simulink model "MPCSimulation"  (R2021b)
settings: Solver=VariableStepAuto  StartTime=0.0  StopTime=tsim  RelTol=1e-3  EnableMultiTasking=on
values from neighbouring files (symbols this model uses):
  C = [eye(4),zeros(4)]    [MPCController.m]    (also in setupsimulation.m)
  M = 3    [MPCController.m]    (also in setupsimulation.m; yalmip_mpc.m)
  Mu = params.l*params.Cfx*eye(nu)    [MPCController.m]    (also in setupsimulation.m)
  Muinv = Mu\eye(nu)    [MPCController.m]    (also in setupsimulation.m)
  Mxi = diag([sqrt(params.Cfx*params.l/params.m),                sqrt(params.Cfx*params.l/params.m),                1,                sqrt(params.Cfx/params.m/params.l)*ones(1,5)])    [MPCController.m]    (also in setupsimulation.m = diag([sqrt(params.Cfx*params.l/params.m),            sqrt(pa)
  Mxinv = Mxi\eye(nx)    [MPCController.m]    (also in setupsimulation.m)
  N = 10    [MPCController.m]    (also in setupsimulation.m; yalmip_mpc.m)
  nu = 4    [MPCController.m]    (also in setupsimulation.m; yalmip_mpc.m)
  nx = 8    [MPCController.m]    (also in setupsimulation.m; yalmip_mpc.m)
  ny = size(C,1)    [MPCController.m]    (also in setupsimulation.m)
  Ts = 0.05    [setupsimulation.m]    (also in yalmip_mpc.m)
  u0 = zeros(4,1)    [setupsimulation.m]
  xi0 = [0; vx0; 0; 0; 250/79*vx0*ones(4,1)]    [setupsimulation.m]
undefined symbols (not defined in the file or in its folder): odeSimulationModel, SimulationModel
settings Model: Creator=johanl  LastModifiedBy=PBM
settings SolverCC: AlgebraicLoopSolver=TrustRegion
settings DataIOCC: LimitDataPoints=on  SaveFormat=Array  SignalLoggingSaveFormat=ModelDataLogs  ReturnWorkspaceOutputs=off
settings OptimizationCC: ExpressionDepthLimit=2147483647  LifeSpan=inf
settings DebuggingCC: UnderspecifiedInitializationDetection=Classic  MergeDetectMultiDrivingBlocksExec=none  SolverPrmCheckMsg=warning  FcnCallInpInsideContextMsg=warning  StateNameClashWarn=warning  SFUnexpectedBacktrackingDiag=warning  SFNoUnconditionalDefaultTransitionDiag=warning  SFExecutionAtInitializationDiag=none  SFMachineParentedDataDiag=warning  ArithmeticOperatorsInVariantConditions=warning
settings HardwareCC: ProdBitPerPointer=32  ProdBitPerSizeT=32  ProdBitPerPtrDiffT=32  ProdLargestAtomicFloat=None  ProdIntDivRoundTo=Undefined  ProdEndianess=Unspecified  ProdWordSize=32  ProdHWDeviceType=32-bit Generic
settings ModelReferenceCC: PropagateSignalLabelsOutOfModel=off
settings SFSimCC: SimUseLocalCustomCode=off  CustomCodeUndefinedFunction=UseInterfaceOnly
settings RTWCC: RTWUseLocalCustomCode=off
settings CodeAppCC: StateflowObjectComments=on
settings GRTTargetCC: TargetLangStandard=C89/C90 (ANSI)
settings ConfigComp: CovMetricSettings=dw  CovSaveCumulativeToWorkspaceVar=on  CovSaveSingleToWorkspaceVar=on  CovExternalEMLEnable=off

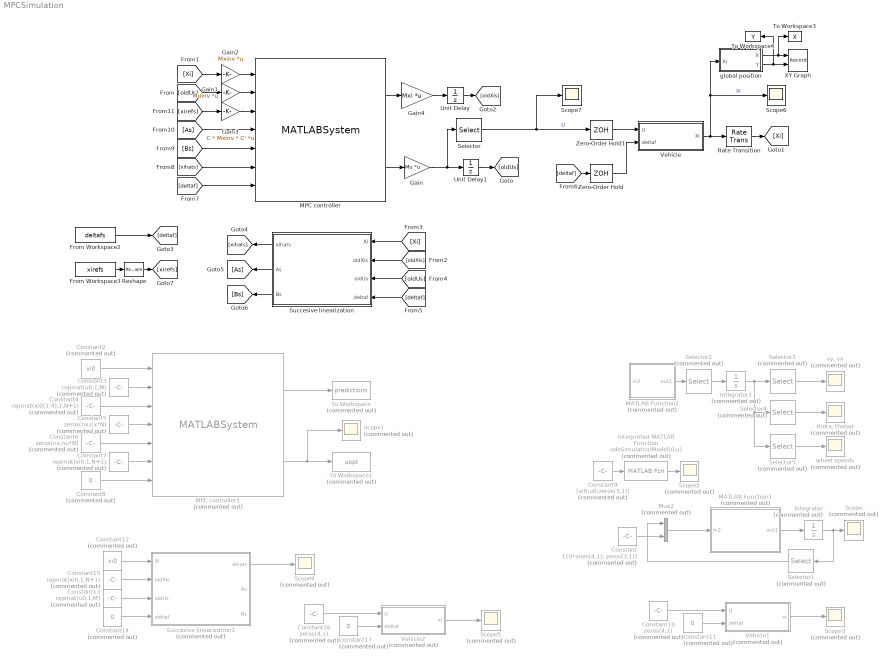
== system MPCSimulation ==
  Constant : Constant  Commented=on  Value=[10*ones(4,1); zeros(3,1)]
  Constant10 : Constant  Commented=on  Value=zeros(4,1)  SampleTime=Ts
  Constant{8,11,14,17} (4 alike) : Constant  Commented=on  Value=0
  Constant12 : Constant  Commented=on  Value=xi0  SampleTime=Ts
  Constant13 : Constant  Commented=on  Value=repmat(u0,1,M)
  Constant15 : Constant  Commented=on  Value=repmat(xi0,1,N+1)
  Constant16 : Constant  Commented=on  Value=zeros(4,1)  SampleTime=Ts
  Constant2 : Constant  Commented=on  Value=xi0  SampleTime=Ts
  Constant3 : Constant  Commented=on  Value=repmat(u0,1,M)
  Constant4 : Constant  Commented=on  Value=repmat(xi0(1:4),1,N+1)
  Constant5 : Constant  Commented=on  Value=zeros(nx,nx*N)
  Constant6 : Constant  Commented=on  Value=zeros(nx,nu*N)
  Constant7 : Constant  Commented=on  Value=repmat(xi0,1,N+1)
  Constant9 : Constant  Commented=on  Value=[xi0;u0;zeros(3,1)]
  From Workspace2 : FromWorkspace  VariableName=deltafs  SampleTime=Ts  OutputAfterFinalValue=Holding final value
  From Workspace3 : FromWorkspace  VariableName=xirefs  SampleTime=Ts  OutputAfterFinalValue=Holding final value
  Gain : Gain  Gain=Mu  Multiplication=Matrix(K*u)
  Gain1 : Gain  Gain=Muinv  Multiplication=Matrix(K*u)
  Gain2 : Gain  Gain=Mxinv  Multiplication=Matrix(K*u)
  Gain3 : Gain  Gain=C * Mxinv * C'  Multiplication=Matrix(K*u)
  Gain4 : Gain  Gain=Mxi  Multiplication=Matrix(K*u)
  Integrator : Integrator  Commented=on  InitialCondition=[0; 10; 0; 0; 250/79*10*ones(4,1);zeros(7,1)];
  Integrator1 : Integrator  Commented=on  InitialCondition=[0; 10; 0; 0; 250/79*10*ones(4,1);zeros(7,1)];
  Interpreted MATLAB Function : MATLABFcn  Commented=on  MATLABFcn=odeSimulationModel(0,u)
  MATLAB Function1 : MATLAB Function  Commented=on  TreatAsAtomicUnit=on
  MATLAB Function2 : MATLAB Function  Commented=on  TreatAsAtomicUnit=on
  MPC controller : MATLABSystem  System=yalmip_mpc  nx=nx  nu=nu  N=N  M=M  Ts=Ts  SimulateUsing=Interpreted execution
      mask Type: yalmip_mpc
      mask Display:
      | disp('yalmip_mpc');
      | port_label('input',1,'Xi');
      | port_label('input',2,'oldUs');
      | port_label('input',3,'xirefs');
      | port_label('input',4,'As');
      | port_label('input',5,'Bs');
      | port_label('input',6,'xihats');
      | port_label('input',7,'deltaf');
      | port_label('output',1,'predictions');
      | port_label('output',2,'uopt');
  MPC controller1 : MATLABSystem  Commented=on  System=yalmip_mpc  nx=nx  nu=nu  N=N  M=M  Ts=Ts  SimulateUsing=Interpreted execution
      mask Type: yalmip_mpc
      mask Display:
      | disp('yalmip_mpc');
      | port_label('input',1,'Xi');
      | port_label('input',2,'oldUs');
      | port_label('input',3,'xirefs');
      | port_label('input',4,'As');
      | port_label('input',5,'Bs');
      | port_label('input',6,'xihats');
      | port_label('input',7,'deltaf');
      | port_label('output',1,'predictions');
      | port_label('output',2,'uopt');
  Mux2 : Mux  Commented=on  Inputs=2
  Rate Transition : RateTransition  InitialCondition=xi0  OutPortSampleTime=Ts
  Reshape : Reshape  OutputDimensionality=Customize  OutputDimensions=[ny,N+1]
  Scope{,1..5} (6 alike) : Scope  Commented=on
  Scope6 : Scope
  Scope7 : Scope
  Selector : Selector  NumberOfDimensions=2  InputPortWidth=3  IndexOptions=Index vector (dialog),Index vector (dialog)  Indices=1:nu,1  OutputSizes=1,1
  Selector1 : Selector  Commented=on  InputPortWidth=15  IndexOptions=Index vector (dialog)  Indices=[1:8]  OutputSizes=1
  Selector2 : Selector  Commented=on  InputPortWidth=15  IndexOptions=Index vector (dialog)  Indices=[1:8]  OutputSizes=1
  Selector3 : Selector  Commented=on  InputPortWidth=8  IndexOptions=Index vector (dialog)  Indices=[1:2]  OutputSizes=1
  Selector4 : Selector  Commented=on  InputPortWidth=8  IndexOptions=Index vector (dialog)  Indices=[3:4]  OutputSizes=1
  Selector5 : Selector  Commented=on  InputPortWidth=8  IndexOptions=Index vector (dialog)  Indices=[5:8]  OutputSizes=1
  Succesive linearization : MATLAB Function  TreatAsAtomicUnit=on
  Succesive linearization1 : MATLAB Function  Commented=on  TreatAsAtomicUnit=on
  To Workspace : ToWorkspace  Commented=on  VariableName=predictions  SaveFormat=Timeseries  SampleTime=-1
  To Workspace1 : ToWorkspace  Commented=on  VariableName=uopt  SaveFormat=Timeseries  SampleTime=-1
  To Workspace3 : ToWorkspace  VariableName=X  SampleTime=-1
  To Workspace4 : ToWorkspace  VariableName=Y  SampleTime=-1
  Unit Delay : UnitDelay  InitialCondition=repmat(xi0,1,N+1)  SampleTime=-1  HasFrameUpgradeWarning=on
  Unit Delay1 : UnitDelay  InitialCondition=repmat(u0,1,M)  SampleTime=-1  HasFrameUpgradeWarning=on
  Vehicle : Subsystem
  Vehicle1 : Subsystem  Commented=on
  Vehicle2 : Subsystem  Commented=on
  XY Graph : Record  FileSettingsInternal="{\"entries\":[{\"content\":{\"excelSettings\":{\"content\":{},\"type\":\"Streamout.ExcelSettings\"}},\"type\":\"Streamout.FileSettingStorage\",\"uuid\":\"9bd8e3e6-cf03-4281-bd11-05e1fe8b1948\"}],\"packageUris\":[\"http://schema.mathworks.com/mf0/streamout_blocks/R2020a\"],\"version\":\"1.0\"}"  Layout=[1 1]  SignalsInternal="{\"entries\":[{\"content\":{\"signals\":[{\"content\":{\"blockPath\":[\"MPCSimulation/XY Graph\"],\"channel\":[],\"dimensions\":[1],\"domain\":\"MPCSimulation/XY Graph\",\"lineColor\":\"#a2142f\",\"plots\":[1],\"port\":1,\"sid\":[],\"signalID\":53,\"signalName\":\"XY Graph:1\"},\"type\":\"RecordBlkView.Signal\",\"uuid\":\"acc0aba6-a077-4c69-b4eb-e56c431fcc30\"},{\"content\":{\"blockPath\":[\"MPCSimulation/XY Graph\"],\"channel\":[],\"dimensions\":[1],\"domain\":\"MPCSimulation/XY Graph\",\"lineColor\":\"#139fff\",\"plots\":[1],\"port\":2,\"sid\":[],\"signalID\":56,\"signalName\":\"XY Graph:2\"},\"type\":\"RecordBlkView.Signal\",\"uuid\":\"2464f634-715d-4349-a932-ac5f9f95b442\"}]},\"type\":\"RecordBlkView.InputSignals\",\"uuid\":\"c07f4d52-6f61-44b7-b332-b508ada1f36c\"}],\"packageUris\":[\"http://schema.mathworks.com/mf0/streamout_blocks/R2020a\"],\"version\":\"1.0\"}"  VisualizationBindings="{\"xyplotplugin\":{\"info\":[{\"series\":[{\"bindingParametersList\":[{\"parameter\":\"X-Axis\",\"signalID\":53,\"signalName\":\"XY Graph:1\"},{\"parameter\":\"Y-Axis\",\"signalID\":56,\"signalName\":\"XY Graph:2\"}],\"seriesID\":48449}],\"subplotID\":1}]}}"  CompatibilityTag=XY  st=-1
  Zero-Order Hold : ZeroOrderHold  SampleTime=Ts
  Zero-Order Hold1 : ZeroOrderHold  SampleTime=Ts
  global position : Subsystem
  "theta, thetad" : Scope  Commented=on
  "vy, vx" : Scope  Commented=on
  wheel speeds : Scope  Commented=on
  wires:
  Integrator1/1 -> Selector5/1, Selector4/1, Selector3/1
  Mux2/1 -> MATLAB Function1/1(in2)
  MATLAB Function1/1(out1) -> Integrator/1
  Integrator/1 -> Selector1/1, Scope/1
  Constant/1 -> Mux2/2
  Selector1/1 -> Mux2/1
  MATLAB Function2/1(out1) -> Selector2/1
  Selector2/1 -> Integrator1/1
  Selector3/1 -> "vy, vx"/1
  Selector4/1 -> "theta, thetad"/1
  Selector5/1 -> wheel speeds/1
  Constant2/1 -> MPC controller1/1
  Constant3/1 -> MPC controller1/2
  Constant4/1 -> MPC controller1/3
  Constant5/1 -> MPC controller1/4
  Constant6/1 -> MPC controller1/5
  Constant7/1 -> MPC controller1/6
  Constant8/1 -> MPC controller1/7
  MPC controller1/1 -> To Workspace/1
  MPC controller1/2 -> Scope1/1, To Workspace1/1
  Constant9/1 -> Interpreted MATLAB Function/1
  Interpreted MATLAB Function/1 -> Scope2/1
  Selector/1 -> Scope7/1, Zero-Order Hold1/1  "U"
  [Xi] -> Gain2/1
  [deltaf] -> Succesive linearization/4(deltaf)
  [deltaf] -> Zero-Order Hold/1
  [deltaf] -> MPC controller/7
  Succesive linearization/1(xihats) -> [xihats]
  Succesive linearization/2(As) -> [As]
  [Bs] -> MPC controller/5
  Succesive linearization/3(Bs) -> [Bs]
  [xihats] -> MPC controller/6
  [As] -> MPC controller/4
  From Workspace2/1 -> [deltaf]
  [xirefs] -> Gain3/1
  Gain/1 -> Unit Delay1/1, Selector/1
  Gain1/1 -> MPC controller/2
  Gain2/1 -> MPC controller/1
  Gain3/1 -> MPC controller/3
  MPC controller/1 -> Gain4/1
  Gain4/1 -> Unit Delay/1
  [oldUs] -> Gain1/1
  MPC controller/2 -> Gain/1
  From Workspace3/1 -> Reshape/1
  Reshape/1 -> [xirefs]
  Constant10/1 -> Vehicle1/1(U)
  Constant11/1 -> Vehicle1/2(deltaf)
  Vehicle1/1(xi) -> Scope3/1
  Constant12/1 -> Succesive linearization1/1(Xi)
  Constant13/1 -> Succesive linearization1/3(oldUs)
  Constant14/1 -> Succesive linearization1/4(deltaf)
  Constant15/1 -> Succesive linearization1/2(oldXis)
  Succesive linearization1/1(xihats) -> Scope4/1
  Vehicle2/1(xi) -> Scope5/1
  Constant17/1 -> Vehicle2/2(deltaf)
  Constant16/1 -> Vehicle2/1(U)
  Vehicle/1(Xi) -> global position/1(Xi), Scope6/1, Rate Transition/1  "Xi"
  Zero-Order Hold/1 -> Vehicle/2(deltaf)
  Zero-Order Hold1/1 -> Vehicle/1(U)
  [Xi] -> Succesive linearization/1(Xi)
  Rate Transition/1 -> [Xi]
  [oldXis] -> Succesive linearization/2(oldXis)
  [oldUs] -> Succesive linearization/3(oldUs)
  Unit Delay1/1 -> [oldUs]
  Unit Delay/1 -> [oldXis]
  global position/1(X) -> To Workspace3/1, XY Graph/1
  global position/2(Y) -> To Workspace4/1, XY Graph/2

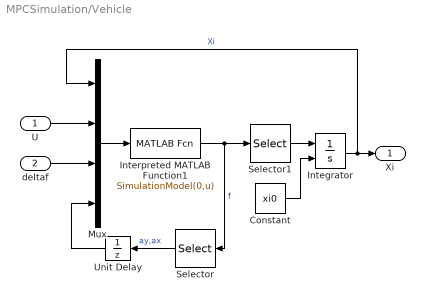
== system MPCSimulation/Vehicle ==
  U : Inport
  deltaf : Inport  Port=2
  Constant : Constant  Value=xi0
  Integrator : Integrator  InitialConditionSource=external  InitialCondition=xi0
  Interpreted MATLAB Function1 : MATLABFcn  MATLABFcn=SimulationModel(0,u)
  Mux : Mux
  Selector : Selector  IndexOptions=Index vector (dialog)  Indices=[1 2]  OutputSizes=1
  Selector1 : Selector  InputPortWidth=15  IndexOptions=Index vector (dialog)  Indices=[1:8]  OutputSizes=1
  Unit Delay : UnitDelay  InitialCondition=[0;0]  SampleTime=-1  HasFrameUpgradeWarning=on
  Xi : Outport  VectorParamsAs1DForOutWhenUnconnected=off
  wires:
  Interpreted MATLAB Function1/1 -> Selector/1, Selector1/1  "f"
  Constant/1 -> Integrator/2
  Integrator/1 -> Mux/1, Xi/1  "Xi"
  Mux/1 -> Interpreted MATLAB Function1/1
  U/1 -> Mux/2
  deltaf/1 -> Mux/3
  Selector1/1 -> Integrator/1
  Selector/1 -> Unit Delay/1  "ay,ax"
  Unit Delay/1 -> Mux/4

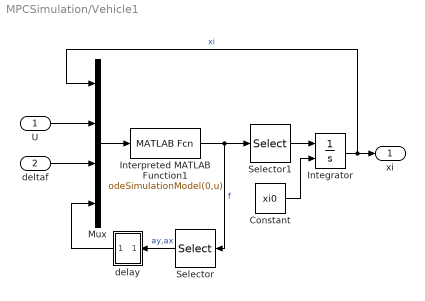
== system MPCSimulation/Vehicle1 ==
  U : Inport
  deltaf : Inport  Port=2
  Constant : Constant  Value=xi0
  Integrator : Integrator  InitialConditionSource=external  InitialCondition=xi0
  Interpreted MATLAB Function1 : MATLABFcn  MATLABFcn=odeSimulationModel(0,u)
  Mux : Mux
  Selector : Selector  IndexOptions=Index vector (dialog)  Indices=[1 2]  OutputSizes=1
  Selector1 : Selector  InputPortWidth=15  IndexOptions=Index vector (dialog)  Indices=[1:8]  OutputSizes=1
  delay : Subsystem
  xi : Outport  VectorParamsAs1DForOutWhenUnconnected=off
  wires:
  Interpreted MATLAB Function1/1 -> Selector/1, Selector1/1  "f"
  Constant/1 -> Integrator/2
  Integrator/1 -> Mux/1, xi/1  "xi"
  Mux/1 -> Interpreted MATLAB Function1/1
  U/1 -> Mux/2
  deltaf/1 -> Mux/3
  Selector1/1 -> Integrator/1
  Selector/1 -> delay/1(" ")  "ay,ax"
  delay/1(Out1) -> Mux/4

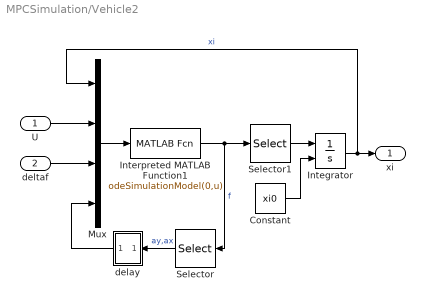
== system MPCSimulation/Vehicle2 ==
  U : Inport
  deltaf : Inport  Port=2
  Constant : Constant  Value=xi0
  Integrator : Integrator  InitialConditionSource=external  InitialCondition=xi0
  Interpreted MATLAB Function1 : MATLABFcn  MATLABFcn=odeSimulationModel(0,u)
  Mux : Mux
  Selector : Selector  IndexOptions=Index vector (dialog)  Indices=[1 2]  OutputSizes=1
  Selector1 : Selector  InputPortWidth=15  IndexOptions=Index vector (dialog)  Indices=[1:8]  OutputSizes=1
  delay : Subsystem
  xi : Outport  VectorParamsAs1DForOutWhenUnconnected=off
  wires:
  Interpreted MATLAB Function1/1 -> Selector/1, Selector1/1  "f"
  Constant/1 -> Integrator/2
  Integrator/1 -> Mux/1, xi/1  "xi"
  Mux/1 -> Interpreted MATLAB Function1/1
  U/1 -> Mux/2
  deltaf/1 -> Mux/3
  Selector1/1 -> Integrator/1
  Selector/1 -> delay/1(" ")  "ay,ax"
  delay/1(Out1) -> Mux/4

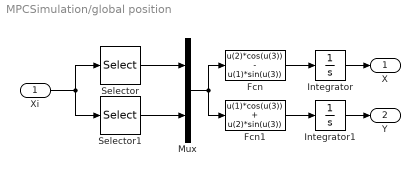
== system MPCSimulation/global position ==
  Xi : Inport
  Fcn : Fcn  Expr=u(2)*cos(u(3)) - u(1)*sin(u(3))
  Fcn1 : Fcn  Expr=u(1)*cos(u(3)) + u(2)*sin(u(3))
  Integrator : Integrator
  Integrator1 : Integrator
  Mux : Mux  Inputs=2
  Selector : Selector  InputPortWidth=8  IndexOptions=Index vector (dialog)  Indices=[1 2]  OutputSizes=1
  Selector1 : Selector  InputPortWidth=8  IndexOptions=Index vector (dialog)  Indices=3  OutputSizes=1
  X : Outport  VectorParamsAs1DForOutWhenUnconnected=off
  Y : Outport  Port=2  VectorParamsAs1DForOutWhenUnconnected=off
  wires:
  Xi/1 -> Selector1/1, Selector/1
  Selector/1 -> Mux/1
  Selector1/1 -> Mux/2
  Fcn/1 -> Integrator/1
  Mux/1 -> Fcn1/1, Fcn/1
  Fcn1/1 -> Integrator1/1
  Integrator/1 -> X/1
  Integrator1/1 -> Y/1

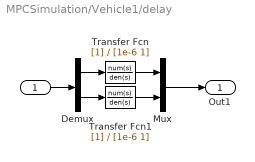
== system MPCSimulation/Vehicle1/delay ==
  " " : Inport
  Demux : Demux  Outputs=2
  Mux : Mux  Inputs=2
  Transfer Fcn : TransferFcn  Denominator=[1e-6 1]
  Transfer Fcn1 : TransferFcn  Denominator=[1e-6 1]
  Out1 : Outport  VectorParamsAs1DForOutWhenUnconnected=off
  wires:
  " "/1 -> Demux/1
  Demux/1 -> Transfer Fcn/1
  Demux/2 -> Transfer Fcn1/1
  Transfer Fcn1/1 -> Mux/2
  Transfer Fcn/1 -> Mux/1
  Mux/1 -> Out1/1

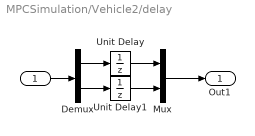
== system MPCSimulation/Vehicle2/delay ==
  " " : Inport
  Demux : Demux  Outputs=2
  Mux : Mux  Inputs=2
  Unit Delay : UnitDelay  SampleTime=-1  HasFrameUpgradeWarning=on
  Unit Delay1 : UnitDelay  SampleTime=-1  HasFrameUpgradeWarning=on
  Out1 : Outport  VectorParamsAs1DForOutWhenUnconnected=off
  wires:
  " "/1 -> Demux/1
  Demux/1 -> Unit Delay/1
  Unit Delay1/1 -> Mux/2
  Unit Delay/1 -> Mux/1
  Mux/1 -> Out1/1
  Demux/2 -> Unit Delay1/1

== matlab function MPCSimulation/MATLAB Function1 ==
  data: in2 input; out1 output
function out1 = odeSimulationModel(in2)
%ODESIMULATIONMODEL
%    OUT1 = ODESIMULATIONMODEL(TS,IN2)

%    This function was generated by the Symbolic Math Toolbox version 8.2.
%    15-Jan-2021 11:04:04

Mp_FL = in2(9,:);
Mp_FR = in2(10,:);
Mp_RL = in2(11,:);
Mp_RR = in2(12,:);
acc_lat_ms2 = in2(14,:);
acc_long_ms2 = in2(15,:);
steer_angle_FL = in2(13,:);
vx = in2(2,:);
vy = in2(1,:);
w_FL = in2(5,:);
w_FR = in2(6,:);
w_RL = in2(7,:);
w_RR = in2(8,:);
yaw_rate = in2(4,:);
t3 = vx.^2;
t6 = acc_lat_ms2.*2.41734219269103e2;
t7 = acc_long_ms2.*1.700046728971963e2;
t8 = t3.*4.29477476635514e-2;
t2 = -t6+t7+t8+3.28635e3;
t77 = yaw_rate.*(3.21e2./2.0e2);
t4 = -t77+vy;
t5 = acc_long_ms2.*5.219143457943925e3;
t9 = t6+t7+t8+3.28635e3;
t10 = t3.*1.318495853271028;
t11 = cos(steer_angle_FL);
t18 = yaw_rate.*7.585e-1;
t12 = -t18+vx;
t13 = t11.*t12;
t14 = sin(steer_angle_FL);
t15 = yaw_rate.*(1.07e2./1.0e2);
t16 = t15+vy;
t17 = t14.*t16;
t19 = t13+t17;
t20 = 1.0./t19;
t39 = w_FL.*(7.9e1./2.5e2);
t21 = t13+t17-t39;
t22 = t18+vx;
t23 = t11.*t22;
t24 = t17+t23;
t25 = 1.0./t24;
t47 = w_FR.*(7.9e1./2.5e2);
t26 = t17+t23-t47;
t27 = acc_lat_ms2.*3.597330257086355e2;
t28 = t7+t8+t27-4.929524999999999e3;
t29 = acc_lat_ms2.*1.104380388925511e4;
t30 = t7+t8-t27-4.929524999999999e3;
t31 = yaw_rate.*(3.01e2./4.0e2);
t32 = t31+vx;
t33 = 1.0./t32;
t62 = w_RR.*(7.9e1./2.5e2);
t34 = t31-t62+vx;
t35 = t31-vx;
t36 = 1.0./t35;
t37 = w_RL.*(7.9e1./2.5e2);
t38 = t31+t37-vx;
t40 = t20.*t21.*3.607731511888605;
t41 = atan(t40);
t42 = t41.*4.0;
t82 = t20.*t21.*1.803865755944303e1;
t43 = t42-t82;
t44 = atan(t43);
t45 = t44.*(2.9e1./2.0e1);
t46 = sin(t45);
t48 = t25.*t26.*3.607731511888605;
t49 = atan(t48);
t50 = t49.*4.0;
t83 = t25.*t26.*1.803865755944303e1;
t51 = t50-t83;
t52 = atan(t51);
t53 = t52.*(2.9e1./2.0e1);
t54 = sin(t53);
t55 = t11.*t16;
t56 = t12.*t14;
t57 = t28.^2;
t58 = t57.*2.35e-3;
t59 = t5+t10+t29+t58-1.513364175e5;
t85 = t14.*t22;
t60 = t55-t85;
t61 = t7+t8-t27-4.929524999999999e3;
t63 = t33.*t34.*3.607731511888605;
t64 = atan(t63);
t65 = t64.*4.0;
t66 = t65-t33.*t34.*1.803865755944303e1;
t67 = atan(t66);
t68 = t67.*(2.9e1./2.0e1);
t69 = sin(t68);
t88 = t36.*t38.*3.607731511888605;
t70 = atan(-t88);
t71 = t70.*4.0;
t72 = t36.*t38.*1.803865755944303e1;
t73 = t71+t72;
t74 = atan(t73);
t75 = t74.*(2.9e1./2.0e1);
t76 = sin(t75);
t78 = acc_lat_ms2.*7.421240531561462e3;
t79 = t2.^2;
t80 = t9.^2;
t81 = t5+t10+t78-t80.*2.35e-3+1.00890945e5;
t84 = t55-t56;
t86 = t7+t8-t27-4.929524999999999e3;
t87 = t7+t8-t27-4.929524999999999e3;
t89 = t2.*t76.*(7.9e1./2.5e2);
t90 = Mp_RL+t89;
out1 = [-vx.*yaw_rate-(t14.*t54.*(t7+t8-t27-4.929524999999999e3))./1.675e3-(t4.*(acc_lat_ms2.*(-7.421240531561462e3)+t5+t10-t79.*2.35e-3+1.00890945e5))./(vx.*1.675e3-yaw_rate.*1.2604375e3)-(t14.*t28.*t46)./1.675e3-(t4.*t33.*t81)./1.675e3+(t11.*t25.*t60.*(t5+t10-t29+t30.^2.*2.35e-3-1.513364175e5))./1.675e3-(t11.*t20.*t59.*(t56-t11.*t16))./1.675e3;t3.*(-2.526268656716418e-4)-(t2.*t76)./1.675e3+(t9.*t69)./1.675e3+vy.*yaw_rate-(t11.*t28.*t46)./1.675e3-(t11.*t30.*t54)./1.675e3-(t14.*t20.*t59.*t84)./1.675e3-(t14.*t25.*t60.*(t5+t10-t29+t61.^2.*2.35e-3-1.513364175e5))./1.675e3;yaw_rate;t2.*t76.*2.875429881543752e-4+t9.*t69.*2.875429881543752e-4+t11.*t28.*t46.*2.898356897210546e-4-t14.*t28.*t46.*4.088651127244937e-4-t11.*t30.*t54.*2.898356897210546e-4-t14.*t30.*t54.*4.088651127244937e-4+t4.*t33.*t81.*6.132976690867405e-4-t4.*t36.*(t5+t10-t78-t79.*2.35e-3+1.00890945e5).*6.132976690867405e-4+t11.*t20.*t59.*t84.*4.088651127244937e-4+t14.*t20.*t59.*t84.*2.898356897210546e-4+t11.*t25.*t60.*(t5+t10-t29+t86.^2.*2.35e-3-1.513364175e5).*4.088651127244937e-4-t14.*t25.*t60.*(t5+t10-t29+t87.^2.*2.35e-3-1.513364175e5).*2.898356897210546e-4;Mp_FL+t28.*t46.*(7.9e1./2.5e2);Mp_FR+t54.*(t7+t8-t27-4.929524999999999e3).*(7.9e1./2.5e2);t90;t90;Mp_FL;Mp_FR;Mp_RL;Mp_RR;steer_angle_FL;acc_lat_ms2;acc_long_ms2];
end

== matlab function MPCSimulation/MATLAB Function2 ==
  data: in2 input; out1 output
function out1 = odeSimulationModel(in2)
%ODESIMULATIONMODEL
%    OUT1 = ODESIMULATIONMODEL(TS,IN2)

%    This function was generated by the Symbolic Math Toolbox version 8.2.
%    15-Jan-2021 11:04:04

Mp_FL = in2(9,:);
Mp_FR = in2(10,:);
Mp_RL = in2(11,:);
Mp_RR = in2(12,:);
acc_lat_ms2 = in2(14,:);
acc_long_ms2 = in2(15,:);
steer_angle_FL = in2(13,:);
vx = in2(2,:);
vy = in2(1,:);
w_FL = in2(5,:);
w_FR = in2(6,:);
w_RL = in2(7,:);
w_RR = in2(8,:);
yaw_rate = in2(4,:);
t3 = vx.^2;
t6 = acc_lat_ms2.*2.41734219269103e2;
t7 = acc_long_ms2.*1.700046728971963e2;
t8 = t3.*4.29477476635514e-2;
t2 = -t6+t7+t8+3.28635e3;
t77 = yaw_rate.*(3.21e2./2.0e2);
t4 = -t77+vy;
t5 = acc_long_ms2.*5.219143457943925e3;
t9 = t6+t7+t8+3.28635e3;
t10 = t3.*1.318495853271028;
t11 = cos(steer_angle_FL);
t18 = yaw_rate.*7.585e-1;
t12 = -t18+vx;
t13 = t11.*t12;
t14 = sin(steer_angle_FL);
t15 = yaw_rate.*(1.07e2./1.0e2);
t16 = t15+vy;
t17 = t14.*t16;
t19 = t13+t17;
t20 = 1.0./t19;
t39 = w_FL.*(7.9e1./2.5e2);
t21 = t13+t17-t39;
t22 = t18+vx;
t23 = t11.*t22;
t24 = t17+t23;
t25 = 1.0./t24;
t47 = w_FR.*(7.9e1./2.5e2);
t26 = t17+t23-t47;
t27 = acc_lat_ms2.*3.597330257086355e2;
t28 = t7+t8+t27-4.929524999999999e3;
t29 = acc_lat_ms2.*1.104380388925511e4;
t30 = t7+t8-t27-4.929524999999999e3;
t31 = yaw_rate.*(3.01e2./4.0e2);
t32 = t31+vx;
t33 = 1.0./t32;
t62 = w_RR.*(7.9e1./2.5e2);
t34 = t31-t62+vx;
t35 = t31-vx;
t36 = 1.0./t35;
t37 = w_RL.*(7.9e1./2.5e2);
t38 = t31+t37-vx;
t40 = t20.*t21.*3.607731511888605;
t41 = atan(t40);
t42 = t41.*4.0;
t82 = t20.*t21.*1.803865755944303e1;
t43 = t42-t82;
t44 = atan(t43);
t45 = t44.*(2.9e1./2.0e1);
t46 = sin(t45);
t48 = t25.*t26.*3.607731511888605;
t49 = atan(t48);
t50 = t49.*4.0;
t83 = t25.*t26.*1.803865755944303e1;
t51 = t50-t83;
t52 = atan(t51);
t53 = t52.*(2.9e1./2.0e1);
t54 = sin(t53);
t55 = t11.*t16;
t56 = t12.*t14;
t57 = t28.^2;
t58 = t57.*2.35e-3;
t59 = t5+t10+t29+t58-1.513364175e5;
t85 = t14.*t22;
t60 = t55-t85;
t61 = t7+t8-t27-4.929524999999999e3;
t63 = t33.*t34.*3.607731511888605;
t64 = atan(t63);
t65 = t64.*4.0;
t66 = t65-t33.*t34.*1.803865755944303e1;
t67 = atan(t66);
t68 = t67.*(2.9e1./2.0e1);
t69 = sin(t68);
t88 = t36.*t38.*3.607731511888605;
t70 = atan(-t88);
t71 = t70.*4.0;
t72 = t36.*t38.*1.803865755944303e1;
t73 = t71+t72;
t74 = atan(t73);
t75 = t74.*(2.9e1./2.0e1);
t76 = sin(t75);
t78 = acc_lat_ms2.*7.421240531561462e3;
t79 = t2.^2;
t80 = t9.^2;
t81 = t5+t10+t78-t80.*2.35e-3+1.00890945e5;
t84 = t55-t56;
t86 = t7+t8-t27-4.929524999999999e3;
t87 = t7+t8-t27-4.929524999999999e3;
t89 = t2.*t76.*(7.9e1./2.5e2);
t90 = Mp_RL+t89;
out1 = [-vx.*yaw_rate-(t14.*t54.*(t7+t8-t27-4.929524999999999e3))./1.675e3-(t4.*(acc_lat_ms2.*(-7.421240531561462e3)+t5+t10-t79.*2.35e-3+1.00890945e5))./(vx.*1.675e3-yaw_rate.*1.2604375e3)-(t14.*t28.*t46)./1.675e3-(t4.*t33.*t81)./1.675e3+(t11.*t25.*t60.*(t5+t10-t29+t30.^2.*2.35e-3-1.513364175e5))./1.675e3-(t11.*t20.*t59.*(t56-t11.*t16))./1.675e3;t3.*(-2.526268656716418e-4)-(t2.*t76)./1.675e3+(t9.*t69)./1.675e3+vy.*yaw_rate-(t11.*t28.*t46)./1.675e3-(t11.*t30.*t54)./1.675e3-(t14.*t20.*t59.*t84)./1.675e3-(t14.*t25.*t60.*(t5+t10-t29+t61.^2.*2.35e-3-1.513364175e5))./1.675e3;yaw_rate;t2.*t76.*2.875429881543752e-4+t9.*t69.*2.875429881543752e-4+t11.*t28.*t46.*2.898356897210546e-4-t14.*t28.*t46.*4.088651127244937e-4-t11.*t30.*t54.*2.898356897210546e-4-t14.*t30.*t54.*4.088651127244937e-4+t4.*t33.*t81.*6.132976690867405e-4-t4.*t36.*(t5+t10-t78-t79.*2.35e-3+1.00890945e5).*6.132976690867405e-4+t11.*t20.*t59.*t84.*4.088651127244937e-4+t14.*t20.*t59.*t84.*2.898356897210546e-4+t11.*t25.*t60.*(t5+t10-t29+t86.^2.*2.35e-3-1.513364175e5).*4.088651127244937e-4-t14.*t25.*t60.*(t5+t10-t29+t87.^2.*2.35e-3-1.513364175e5).*2.898356897210546e-4;Mp_FL+t28.*t46.*(7.9e1./2.5e2);Mp_FR+t54.*(t7+t8-t27-4.929524999999999e3).*(7.9e1./2.5e2);t90;t90;Mp_FL;Mp_FR;Mp_RL;Mp_RR;steer_angle_FL;acc_lat_ms2;acc_long_ms2];
end

== matlab function MPCSimulation/Succesive linearization ==
  settings: updateMethod=DISCRETE  sampleTime=Ts
  data: Xi input; xihats output; oldXis input; oldUs input; deltaf input; As output; Bs output; MPCData parameter
function [xihats,As,Bs] = fcn(Xi,oldXis,oldUs,deltaf,MPCData)
N = MPCData.N;
M = MPCData.M;
nx = MPCData.nx;
nu = MPCData.nu;

Mxi = MPCData.Mxi;
Mxinv = MPCData.Mxinv;
Mu = MPCData.Mu;
that = MPCData.that;
Ts = MPCData.Ts;
Tsp = MPCData.Tsp;

xihats = nan(nx,N+1);
As = nan(nx,nx*N);
Bs = nan(nx,nu*N);
xihat = Xi;
xihats(:,1) = Mxinv * Xi;
for j = 1:N
    if j > M
        [~,xihat] = ode45(@OdeTwoTrackModel,[0,Ts],[xihat;oldUs(:,M);deltaf]);
        [A,B] = TwoTrackModelJacobian(oldXis(:,j),oldUs(:,M),deltaf);
    else
        [~,xihat] = ode45(@OdeTwoTrackModel,[0,Ts],[xihat;oldUs(:,j);deltaf]);
        [A,B] = TwoTrackModelJacobian(oldXis(:,j),oldUs(:,j),deltaf);
    end
    xihat = xihat(end,1:8)';  % nx*(N+1)
    % transform to Pi-space
    xihats(:,j+1) = Mxinv * xihat;

    % formulate in Pi-space and discretize (from c2d.m)
    Ap = that * Mxinv * A * Mxi;
    Bp = that * Mxinv * B * Mu;
    [~,n] = size(Ap);
    [~,nb] = size(Bp);
    s = expm([[Ap Bp]*Ts; zeros(nb,n+nb)]);
    Ad = s(1:n,1:n);
    Bd= s(1:n,n+1:n+nb);
    
    As(:,nx*(j-1)+1:nx*j) = Ad;
    Bs(:,nu*(j-1)+1:nu*j) = Bd;       
end

== matlab function MPCSimulation/Succesive linearization1 ==
  data: Xi input; xihats output; oldXis input; oldUs input; deltaf input; As output; Bs output; MPCData parameter
function [xihats,As,Bs] = fcn(Xi,oldXis,oldUs,deltaf,MPCData)
N = MPCData.N;
M = MPCData.M;
nx = MPCData.nx;
nu = MPCData.nu;

% enablePi = 1;
% Mxi = diag([sqrt(params.Cfx*params.l/params.m),...
%            sqrt(params.Cfx*params.l/params.m),...
%            1,...
%            sqrt(params.Cfx/params.m/params.l)*ones(1,5)]);
% if ~enablePi; Mxi = eye(8); end
% Mxinv = Mxi\eye(nx);
% Mu = params.l*params.Cfx*eye(nu);
% if ~enablePi; Mu = eye(4); end
% %Muinv = Mu\eye(nu);
% that = sqrt(params.m*params.l/params.Cfx);  % time conversion factor t=that*tp
% if ~enablePi; that = 1; end
% Tsp = Ts/that;  % normalize time units

Mxi = MPCData.Mxi;
Mxinv = MPCData.Mxinv;
Mu = MPCData.Mu;
that = MPCData.that;
Ts = MPCData.Ts;
Tsp = MPCData.Tsp;

xihats = nan(nx,N+1);
As = nan(nx,nx*N);
Bs = nan(nx,nu*N);
xihat = Xi;
xihats(:,1) = Mxinv * Xi;
for j = 1:N
    if j > M
        [~,xihat] = ode45(@odeTwoTrackModel,[0,Ts],[xihat;oldUs(:,M);deltaf]);
        [A,B] = twoTrackModelJacobian(oldXis(:,j),oldUs(:,M),deltaf);
    else
        [~,xihat] = ode45(@odeTwoTrackModel,[0,Ts],[xihat;oldUs(:,j);deltaf]);
        [A,B] = twoTrackModelJacobian(oldXis(:,j),oldUs(:,j),deltaf);
    end
    xihat = xihat(end,1:8)';  % nx*(N+1)
    % transform to Pi-space
    xihats(:,j+1) = Mxinv * xihat;

    % formulate in Pi-space and discretize
    Ap = that * Mxinv * A * Mxi;
    Bp = that * Mxinv * B * Mu;
%     [Ad,Bd] = c2d(Ap,Bp,Tsp);
    [m,n] = size(Ap); %#ok<ASGLU>
    [m,nb] = size(Bp); %#ok<ASGLU>
    s = expm([[Ap Bp]*Ts; zeros(nb,n+nb)]);
    Ad = s(1:n,1:n);
    Bd= s(1:n,n+1:n+nb);
    
    As(:,nx*(j-1)+1:nx*j) = Ad;
    Bs(:,nu*(j-1)+1:nu*j) = Bd;       
end
